simulink model "simiam_demo"  (Simulink 8.0)
settings: Solver=ode45  StartTime=0.0  StopTime=10.0  RelTol=1e-3
libraries: simiam x1
settings Model: Creator=jdelacroix  LastModifiedBy=jdelacroix
settings DataIOCC: SignalLoggingSaveFormat=ModelDataLogs
settings DebuggingCC: FcnCallInpInsideContextMsg=EnableAllAsWarning

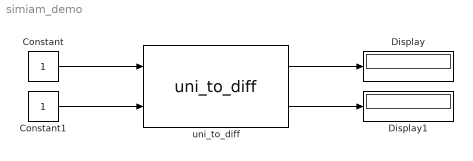
== system simiam_demo ==
  Constant : Constant
  Constant1 : Constant
  Display : Display
  Display1 : Display
  uni_to_diff : simiam/uni_to_diff  wheel_radius=0.021  wheel_base_length=0.0885
  wires:
  uni_to_diff/2 -> Display1/1
  uni_to_diff/1 -> Display/1
  Constant/1 -> uni_to_diff/1
  Constant1/1 -> uni_to_diff/2
